simulink model "SOFC"  (R2016b)
settings: Solver=ode45  StartTime=0.0  StopTime=time  MaxStep=1.0  RelTol=1e-3
values from neighbouring files (symbols this model uses):
  I_fc = I_pattern(k)    [Model_based_FDI.m]    (also in SOFC_Model.m; model_valid.m)
  N = 384    [Model_based_FDI.m]    (also in SOFC_Model.m; model_valid.m = 30)
  qin_H2 = qin_H2_standard    (= 2.4)    [Model_based_FDI.m]    (also in SOFC_Model.m = qin_H2_standard*lossrate; model_valid.m)
  R_HO = R_HO_standard    (= 1.144)    [Model_based_FDI.m]    (also in SOFC_Model.m; model_valid.m)
  T_fc = 1375    [Model_based_FDI.m]    (also in SOFC_Model.m; model_valid.m)
  Tao_H2 = 26.1    [Model_based_FDI.m]    (also in SOFC_Model.m; model_valid.m)
  Tao_H2O = 78.3    [Model_based_FDI.m]    (also in SOFC_Model.m; model_valid.m)
  Tao_O2 = 2.91    [Model_based_FDI.m]    (also in SOFC_Model.m; model_valid.m)
settings Model: Creator=LWL  LastModifiedBy=LWL

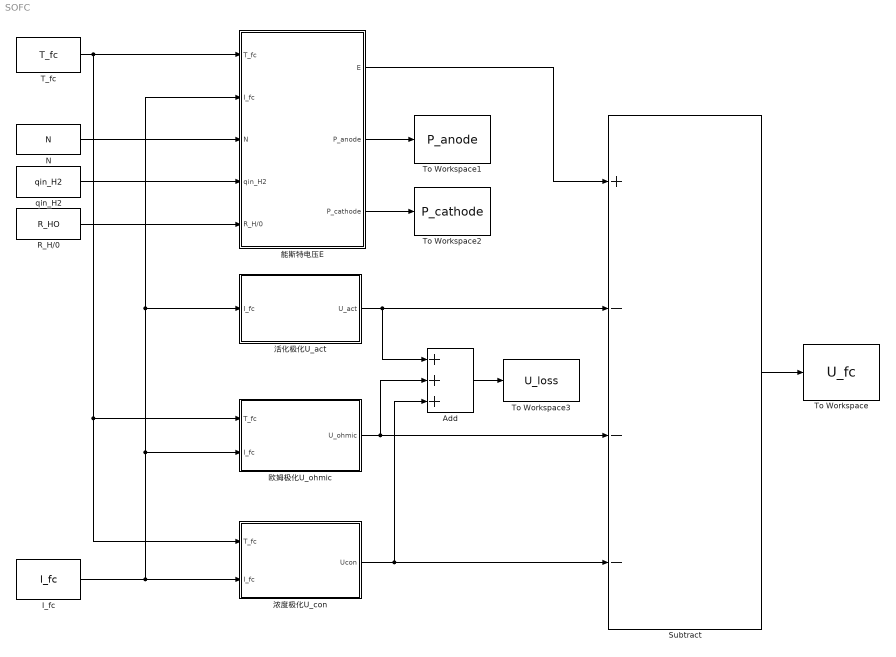
== system SOFC ==
  Add : Sum  Inputs=+++
  I_fc : Constant  Value=I_fc
  N : Constant  Value=N
  R_H/0 : Constant  Value=R_HO
  Subtract : Sum  Inputs=+---
  T_fc : Constant  Value=T_fc
  To Workspace : ToWorkspace  VariableName=U_fc  SaveFormat=Timeseries  SampleTime=-1
  To Workspace1 : ToWorkspace  VariableName=P_anode  SaveFormat=Timeseries  SampleTime=-1
  To Workspace2 : ToWorkspace  VariableName=P_cathode  SaveFormat=Timeseries  SampleTime=-1
  To Workspace3 : ToWorkspace  VariableName=U_loss  SaveFormat=Timeseries  SampleTime=-1
  qin_H2 : Constant  Value=qin_H2
  欧姆极化U_ohmic : Subsystem
  活化极化U_act : Subsystem
  浓度极化U_con : Subsystem
  能斯特电压E : Subsystem
  wires:
  T_fc/1 -> 浓度极化U_con/1(T_fc), 欧姆极化U_ohmic/1(T_fc), 能斯特电压E/1(T_fc)
  I_fc/1 -> 能斯特电压E/2("I_fc "), 活化极化U_act/1(I_fc), 欧姆极化U_ohmic/2(I_fc), 浓度极化U_con/2("I_fc ")
  活化极化U_act/1("U_act ") -> Add/1, Subtract/2
  欧姆极化U_ohmic/1(U_ohmic) -> Subtract/3, Add/2
  浓度极化U_con/1(Ucon) -> Add/3, Subtract/4
  Subtract/1 -> To Workspace/1
  N/1 -> 能斯特电压E/3(N)
  qin_H2/1 -> 能斯特电压E/4(qin_H2)
  R_H/0/1 -> 能斯特电压E/5(R_H/0)
  能斯特电压E/1(E) -> Subtract/1
  能斯特电压E/2(P_anode) -> To Workspace1/1
  能斯特电压E/3(P_cathode) -> To Workspace2/1
  Add/1 -> To Workspace3/1

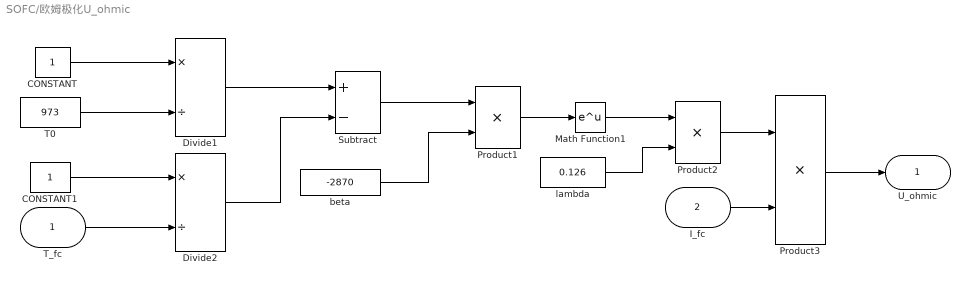
== system SOFC/欧姆极化U_ohmic ==
  T_fc : Inport
  I_fc : Inport  Port=2
  CONSTANT : Constant
  CONSTANT1 : Constant
  Divide1 : Product  Inputs=*/
  Divide2 : Product  Inputs=*/
  Math Function1 : Math  SaturateOnIntegerOverflow=on
  Product1 : Product
  Product2 : Product
  Product3 : Product
  Subtract : Sum  Inputs=+-
  "T0 " : Constant  Value=973
  beta : Constant  Value=-2870
  lambda : Constant  Value=0.126
  U_ohmic : Outport
  wires:
  Subtract/1 -> Product1/1
  CONSTANT1/1 -> Divide2/1
  beta/1 -> Product1/2
  "T0 "/1 -> Divide1/2
  T_fc/1 -> Divide2/2
  Divide2/1 -> Subtract/2
  CONSTANT/1 -> Divide1/1
  Product1/1 -> Math Function1/1
  lambda/1 -> Product2/2
  Math Function1/1 -> Product2/1
  I_fc/1 -> Product3/2
  Product2/1 -> Product3/1
  Divide1/1 -> Subtract/1
  Product3/1 -> U_ohmic/1

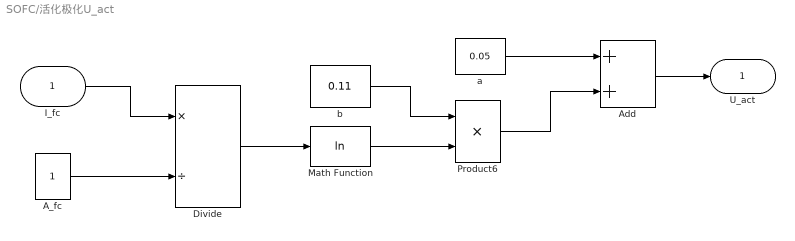
== system SOFC/活化极化U_act ==
  I_fc : Inport
  A_fc : Constant
  Add : Sum
  Divide : Product  Inputs=*/
  Math Function : Math  Operator=log  SaturateOnIntegerOverflow=on
  Product6 : Product
  a : Constant  Value=0.05
  b : Constant  Value=0.11
  "U_act " : Outport
  wires:
  A_fc/1 -> Divide/2
  Math Function/1 -> Product6/2
  Add/1 -> "U_act "/1
  Product6/1 -> Add/2
  I_fc/1 -> Divide/1
  b/1 -> Product6/1
  a/1 -> Add/1
  Divide/1 -> Math Function/1

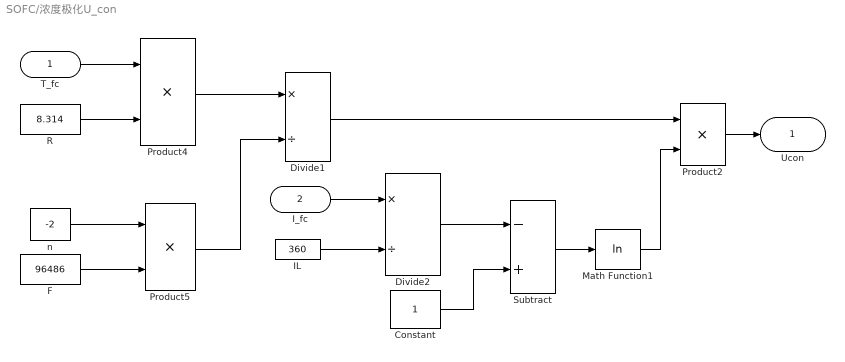
== system SOFC/浓度极化U_con ==
  T_fc : Inport
  "I_fc " : Inport  Port=2
  Constant : Constant
  Divide1 : Product  Inputs=*/
  Divide2 : Product  Inputs=*/
  F : Constant  Value=96486
  IL : Constant  Value=360
  Math Function1 : Math  Operator=log  SaturateOnIntegerOverflow=on
  Product2 : Product
  Product4 : Product
  Product5 : Product
  "R " : Constant  Value=8.314
  Subtract : Sum  Inputs=-+
  n : Constant  Value=-2
  Ucon : Outport
  wires:
  Product2/1 -> Ucon/1
  Product5/1 -> Divide1/2
  Product4/1 -> Divide1/1
  T_fc/1 -> Product4/1
  F/1 -> Product5/2
  IL/1 -> Divide2/2
  n/1 -> Product5/1
  Divide2/1 -> Subtract/1
  Subtract/1 -> Math Function1/1
  "R "/1 -> Product4/2
  "I_fc "/1 -> Divide2/1
  Divide1/1 -> Product2/1
  Constant/1 -> Subtract/2
  Math Function1/1 -> Product2/2

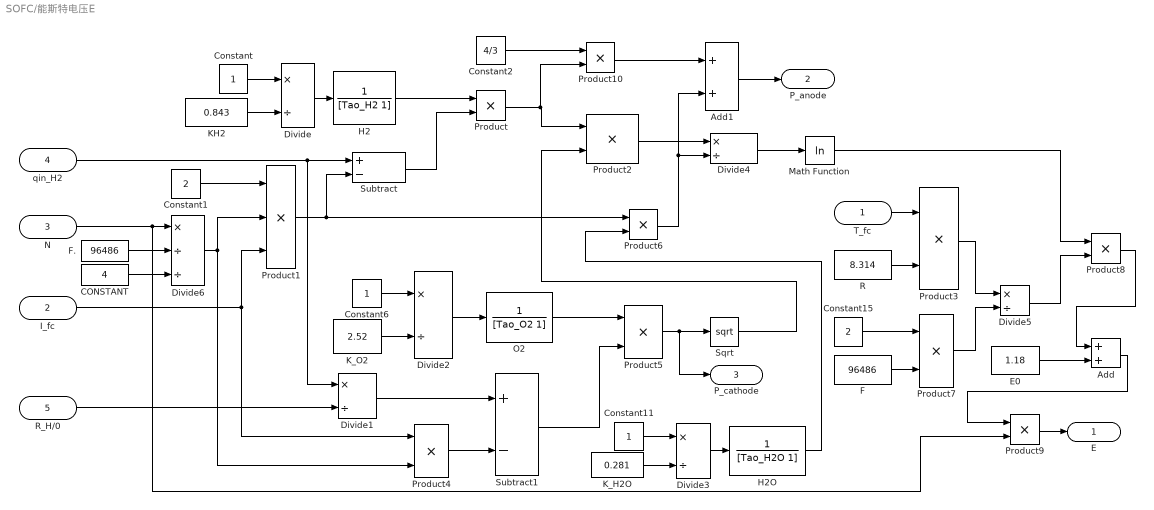
== system SOFC/能斯特电压E ==
  T_fc : Inport
  "I_fc " : Inport  Port=2
  N : Inport  Port=3
  qin_H2 : Inport  Port=4
  R_H/0 : Inport  Port=5
  Add : Sum
  Add1 : Sum
  "CONSTANT " : Constant  Value=4
  Constant : Constant
  Constant1 : Constant  Value=2
  Constant11 : Constant
  Constant15 : Constant  Value=2
  Constant2 : Constant  Value=4/3
  Constant6 : Constant
  Divide{,1..5} (6 alike) : Product  Inputs=*/
  Divide6 : Product  Inputs=*//
  E0 : Constant  Value=1.18
  F : Constant  Value=96486
  F. : Constant  Value=96486
  H2 : TransferFcn  Denominator=[Tao_H2 1]
  H2O : TransferFcn  Denominator=[Tao_H2O 1]
  "KH2 " : Constant  Value=0.843
  "K_H2O " : Constant  Value=0.281
  "K_O2 " : Constant  Value=2.52
  Math Function : Math  Operator=log  SaturateOnIntegerOverflow=on
  O2 : TransferFcn  Denominator=[Tao_O2 1]
  Product{,2..10} (10 alike) : Product
  Product1 : Product  Inputs=3
  R : Constant  Value=8.314
  Sqrt : Sqrt  SaturateOnIntegerOverflow=on
  Subtract : Sum  Inputs=+-
  Subtract1 : Sum  Inputs=+-
  E : Outport
  P_anode : Outport  Port=2
  P_cathode : Outport  Port=3
  wires:
  H2/1 -> Product/1
  Product1/1 -> Product6/1, Subtract/2
  Product2/1 -> Divide4/1
  Divide/1 -> H2/1
  Constant1/1 -> Product1/1
  Divide2/1 -> O2/1
  Product4/1 -> Subtract1/2
  Product5/1 -> P_cathode/1, Sqrt/1
  Sqrt/1 -> Product2/2
  Subtract/1 -> Product/2
  Constant/1 -> Divide/1
  Divide4/1 -> Math Function/1
  Divide1/1 -> Subtract1/1
  Subtract1/1 -> Product5/2
  Product/1 -> Product10/2, Product2/1
  O2/1 -> Product5/1
  Constant6/1 -> Divide2/1
  "K_O2 "/1 -> Divide2/2
  "KH2 "/1 -> Divide/2
  "I_fc "/1 -> Product1/3, Product4/1
  "K_H2O "/1 -> Divide3/2
  Divide3/1 -> H2O/1
  Constant11/1 -> Divide3/1
  Product8/1 -> Add/1
  Math Function/1 -> Product8/1
  E0/1 -> Add/2
  Constant15/1 -> Product7/1
  Add/1 -> Product9/1
  Product6/1 -> Add1/2, Divide4/2
  R/1 -> Product3/2
  Product7/1 -> Divide5/2
  Divide5/1 -> Product8/2
  Product3/1 -> Divide5/1
  H2O/1 -> Product6/2
  F/1 -> Product7/2
  T_fc/1 -> Product3/1
  Product9/1 -> E/1
  N/1 -> Divide6/1, Product9/2
  Divide6/1 -> Product4/2, Product1/2
  F./1 -> Divide6/2
  "CONSTANT "/1 -> Divide6/3
  qin_H2/1 -> Divide1/1, Subtract/1
  R_H/0/1 -> Divide1/2
  Constant2/1 -> Product10/1
  Product10/1 -> Add1/1
  Add1/1 -> P_anode/1
